simulink model "COMPARE_ODE_Solvers_sim"  (R2019b)
settings: Solver=ode8  StartTime=0  StopTime=2*pi  FixedStep=pi/100  RelTol=1e-6  EnableMultiTasking=on
settings Model: Creator=David  LastModifiedBy=sulaymon.eshkabilov
settings DataIOCC: ExternalInput=[t, t]  LimitDataPoints=on  SaveFormat=Array  SignalLoggingSaveFormat=ModelDataLogs  ReturnWorkspaceOutputs=off
settings OptimizationCC: ExpressionDepthLimit=2147483647  LifeSpan=inf
settings DebuggingCC: UnderspecifiedInitializationDetection=Classic  MergeDetectMultiDrivingBlocksExec=none  SolverPrmCheckMsg=warning  FcnCallInpInsideContextMsg=warning  StateNameClashWarn=warning  SFUnexpectedBacktrackingDiag=warning  SFNoUnconditionalDefaultTransitionDiag=warning  SFExecutionAtInitializationDiag=none  ArithmeticOperatorsInVariantConditions=warning
settings HardwareCC: ProdBitPerPointer=32  ProdBitPerSizeT=32  ProdBitPerPtrDiffT=32  ProdLargestAtomicFloat=None  ProdIntDivRoundTo=Undefined  ProdEndianess=Unspecified  ProdWordSize=32  ProdHWDeviceType=32-bit Generic
settings ModelReferenceCC: PropagateSignalLabelsOutOfModel=off
settings SFSimCC: SimUseLocalCustomCode=off  CustomCodeUndefinedFunction=UseInterfaceOnly
settings RTWCC: RTWUseLocalCustomCode=off
settings CodeAppCC: StateflowObjectComments=on
settings GRTTargetCC: TargetLangStandard=C89/C90 (ANSI)  GeneratePreprocessorConditionals=Disable all  CombineOutputUpdateFcns=off  GRTInterface=on
settings ConfigComp: CovMetricSettings=dw  CovHtmlReporting=on  CovSaveCumulativeToWorkspaceVar=on  CovSaveSingleToWorkspaceVar=on  CovExternalEMLEnable=off

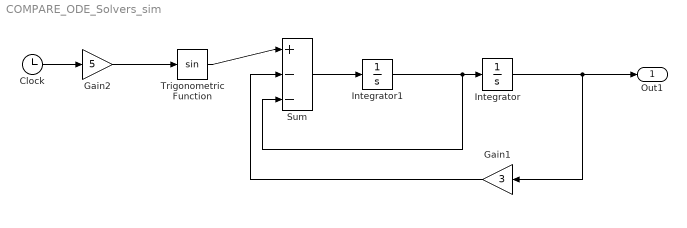
== system COMPARE_ODE_Solvers_sim ==
  Clock : Clock
  Gain1 : Gain  Gain=3
  Gain2 : Gain  Gain=5
  Integrator : Integrator  InitialCondition=3
  Integrator1 : Integrator  InitialCondition=-2
  Sum : Sum  Inputs=|+--
  Trigonometric Function : Trigonometry
  Out1 : Outport
  wires:
  Clock/1 -> Gain2/1
  Gain2/1 -> Trigonometric Function/1
  Sum/1 -> Integrator1/1
  Integrator1/1 -> Integrator/1, Sum/3
  Integrator/1 -> Out1/1, Gain1/1
  Gain1/1 -> Sum/2
  Trigonometric Function/1 -> Sum/1
